simulink model "RosPubSubExample"  (Simulink 9.1)
settings: Solver=FixedStepAuto  StartTime=0.0  StopTime=10.0  FixedStep=0.01  RelTol=1e-3
libraries: RosToolbox x2
settings Model: SuppressorTable=22 serialization::archive 11 0 6 0 0 0 1 0  Creator=dferigo  LastModifiedBy=dferigo
settings DataIOCC: SaveFormat=Dataset
settings OptimizationCC: LifeSpan=auto
settings DebuggingCC: UnderspecifiedInitializationDetection=Simplified  MergeDetectMultiDrivingBlocksExec=error  SFUnexpectedBacktrackingDiag=error  SFNoUnconditionalDefaultTransitionDiag=error  SFExecutionAtInitializationDiag=warning
settings HardwareCC: ProdBitPerPointer=64  ProdBitPerSizeT=64  ProdBitPerPtrDiffT=64  ProdLargestAtomicFloat=Float  ProdIntDivRoundTo=Zero  ProdEndianess=LittleEndian  ProdWordSize=64  ProdHWDeviceType=Intel->x86-64 (Windows64)
settings ModelReferenceCC: PropagateSignalLabelsOutOfModel=on
settings RTWCC: GenCodeOnly=on  TargetLang=C++
settings CodeAppCC: StateflowObjectComments=off
settings GRTTargetCC: TargetLangStandard=C++03 (ISO)  CombineOutputUpdateFcns=on  MatFileLogging=off  MultiInstanceERTCode=on  CodeInterfacePackaging=C++ class  GRTInterface=off
settings CPPComponent: GenerateDestructor=on  GenerateExternalIOAccessMethods=None  ParameterMemberVisibility=private  InternalMemberVisibility=private  GenerateParameterAccessMethods=None  GenerateInternalMemberAccessMethods=None  UseOperatorNewForModelRefRegistration=off
settings ConfigComp: CovMetricSettings=dwe  CovHtmlReporting=off  CovSaveCumulativeToWorkspaceVar=off  CovSaveSingleToWorkspaceVar=off  CovExternalEMLEnable=on

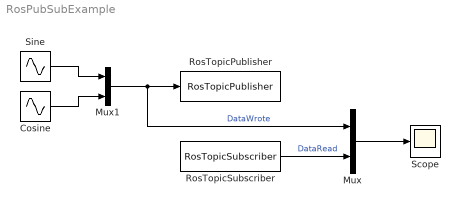
== system RosPubSubExample ==
  Cosine : Sin  Phase=pi/2  SampleTime=0
  Mux : Mux  Inputs=2
  Mux1 : Mux  Inputs=2
  RosTopicPublisher : RosToolbox/RosTopicPublisher  TopicName=/PubSubExample  QueueSize=1
      settings: SourceProductName=Ros Toolbox
  RosTopicSubscriber : RosToolbox/RosTopicSubscriber  TopicName=/PubSubExample  MessageSize=2
      settings: SourceProductName=Ros Toolbox
  Scope : Scope
  Sine : Sin  SampleTime=0
  wires:
  Mux1/1 -> RosTopicPublisher/1, Mux/1  "DataWrote"
  Mux/1 -> Scope/1
  RosTopicSubscriber/1 -> Mux/2  "DataRead"
  Sine/1 -> Mux1/1
  Cosine/1 -> Mux1/2
